simulink model "Turbine_PSI_TestBed_org"  (Simulink 10.0)
settings: Solver=FixedStepDiscrete  StartTime=0.0  StopTime=1  FixedStep=1  RelTol=1e-3  EnableMultiTasking=on
undefined symbols (not defined in the file): MWS
libraries: Lib_Turbo_TurbinePSI_TMATS x1
settings Model: Creator=jwchapm2  LastModifiedBy=annonymous
settings DataIOCC: LimitDataPoints=on
settings OptimizationCC: ExpressionDepthLimit=2147483647
settings DebuggingCC: SolverPrmCheckMsg=warning  StateNameClashWarn=warning
settings GRTTargetCC: GeneratePreprocessorConditionals=Disable all  CombineOutputUpdateFcns=on  GRTInterface=off
settings ConfigComp: CovExternalEMLEnable=off

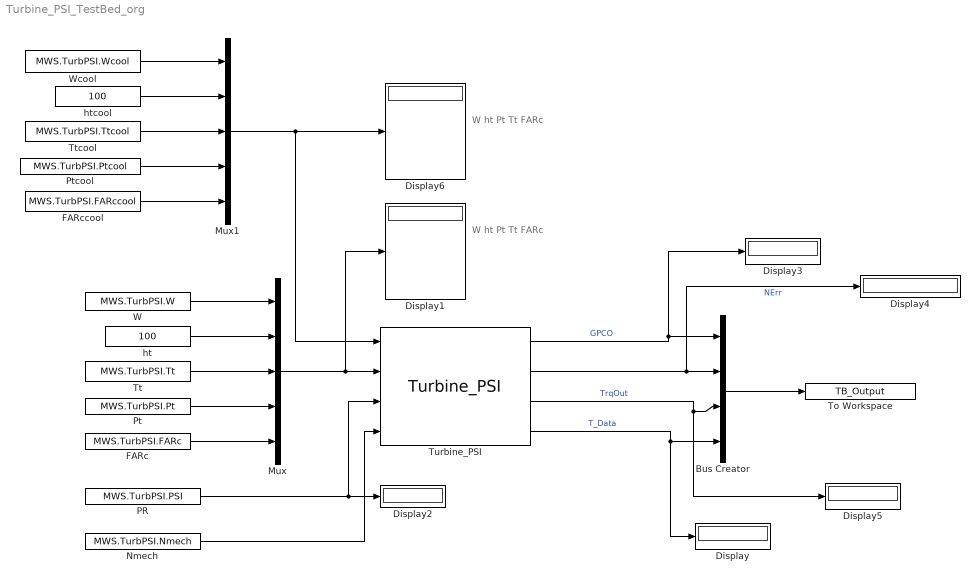
== system Turbine_PSI_TestBed_org ==
  note: W
      | ht
      | Pt
      | Tt
      | FARc
  note: W
      | ht
      | Pt
      | Tt
      | FARc
  Bus Creator : BusCreator  Inputs=4
  Display{,1..6} (7 alike) : Display
  FARc : Constant  Value=MWS.TurbPSI.FARc
  FARccool : Constant  Value=MWS.TurbPSI.FARccool
  Mux : Mux  Inputs=5
  Mux1 : Mux  Inputs=5
  Nmech : Constant  Value=MWS.TurbPSI.Nmech
  PR : Constant  Value=MWS.TurbPSI.PSI
  Pt : Constant  Value=MWS.TurbPSI.Pt
  Ptcool : Constant  Value=MWS.TurbPSI.Ptcool
  To Workspace : ToWorkspace  VariableName=TB_Output  SampleTime=-1
  Tt : Constant  Value=MWS.TurbPSI.Tt
  Ttcool : Constant  Value=MWS.TurbPSI.Ttcool
  Turbine_PSI : Lib_Turbo_TurbinePSI_TMATS/Turbine_PSI  X_T_PRpVec_M=MWS.TurbPSI.PRVec  Y_T_NcpVec_M=MWS.TurbPSI.NcVec  T_T_Map_PSIArray_M=MWS.TurbPSI.PSIArrayI  X_T_PRwVec_M=MWS.TurbPSI.PRVec  Y_T_NcwVec_M=MWS.TurbPSI.NcVec  T_T_Map_WoWArray_M=MWS.TurbPSI.WoWArray  s_T_hi_M=MWS.TurbPSI.hi  s_T_Nc_M=MWS.TurbPSI.s_Nc  s_T_PR_M=MWS.TurbPSI.s_PR  s_T_Wc_M=MWS.TurbPSI.s_Wc  s_T_Eff_M=MWS.TurbPSI.s_eff  CFlwEn_M=on  T_CoolFlwPos_M=MWS.TurbPSI.CF  gamma_M=1.4  Rt_M=0.1  iDesign_M=off  NcDes_M=100  EffDes_M=0.9328  PRDes_M=5  NDes_M=10000
  W : Constant  Value=MWS.TurbPSI.W
  Wcool : Constant  Value=MWS.TurbPSI.Wcool
  ht : Constant  Value=100
  htcool : Constant  Value=100
  wires:
  PR/1 -> Turbine_PSI/3, Display2/1
  W/1 -> Mux/1
  FARc/1 -> Mux/5
  Tt/1 -> Mux/3
  Pt/1 -> Mux/4
  Mux/1 -> Turbine_PSI/2, Display1/1
  Turbine_PSI/1 -> Bus Creator/1, Display3/1  "GPCO"
  Turbine_PSI/2 -> Bus Creator/2, Display4/1  "NErr"
  Turbine_PSI/3 -> Bus Creator/3, Display5/1  "TrqOut"
  Turbine_PSI/4 -> Display/1, Bus Creator/4  "T_Data"
  Bus Creator/1 -> To Workspace/1
  ht/1 -> Mux/2
  Nmech/1 -> Turbine_PSI/4
  Wcool/1 -> Mux1/1
  FARccool/1 -> Mux1/5
  Ttcool/1 -> Mux1/3
  Ptcool/1 -> Mux1/4
  Mux1/1 -> Turbine_PSI/1, Display6/1
  htcool/1 -> Mux1/2
